simulink model "AttitudeControlSim"  (R2024b)
settings: Solver=VariableStepAuto  StartTime=0.0  StopTime=1000  RelTol=1e-3
values from neighbouring files (symbols this model uses):
  A = RWSConfig(beta)    [RWSTiltAngleOptimisation.m]
  Js = 0.001    [RWSTiltAngleOptimisation.m]
  Kd = diag([20;20;24])    [RWSTiltAngleOptimisation.m]
  Kp = diag([10;10;12])    [RWSTiltAngleOptimisation.m]
  omega0 = 0    [RWSTiltAngleOptimisation.m]
undefined symbols (not defined in the file or in its folder): orb, sat
libraries: aerolibutil x3, matrix_library x2, sharedutil x1
settings Model: PacingRate=2  Creator=Ameya  LastModifiedBy=Ameya

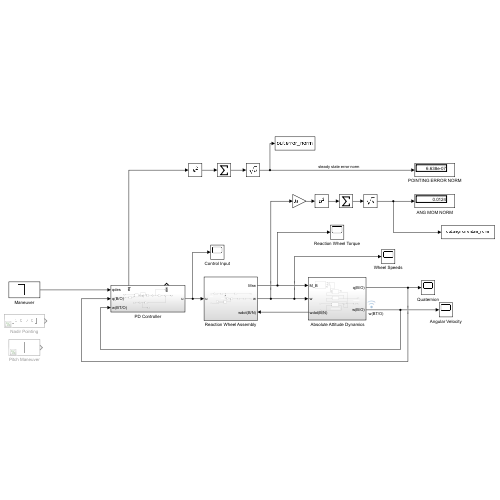
[thumbnail: Simulink's stored preview of the top-level diagram]
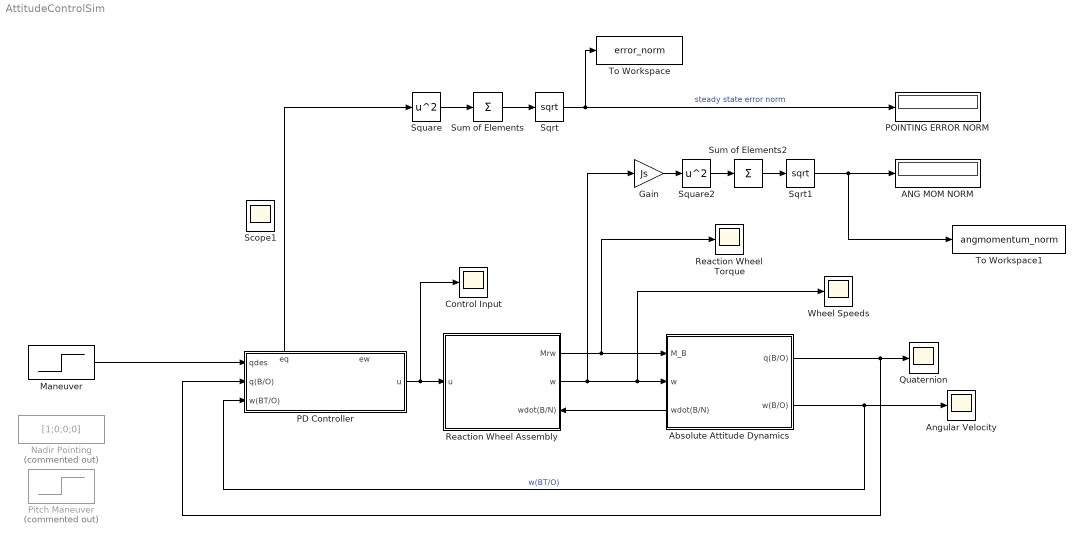
== system AttitudeControlSim ==
  " Absolute Attitude Dynamics" : Subsystem
      settings: PortSchema="{\"entries\":[{\"content\":{\"sides\":[{\"content\":{\"connectorIds\":[\"In1\",\"In2\",\"Out3\"]},\"type\":\"ConnectorPlacement.EquallySpacedRectSide\",\"uuid\":\"5cc1fa62-5eb8-4e37-8643-9896299a6aa0\"},{\"content\":{\"connectorIds\":[\"Out1\",\"Out2\"],\"side\":\"RIGHT\"},\"type\":\"ConnectorPlacement.EquallySpacedRectSide\",\"uuid\":\"f1722523-4fb3-4755-a040-6e35a0c45818\"},{\"content\":{\"side\":\"TOP\"},\"type\":\"ConnectorPlacement.EquallySpacedRectSide\",\"uuid\":\"c8585ddf-0cc3-42b7-bd60-482c1818a7a4\"}]},\"type\":\"ConnectorPlacement.EquallySpacedConnector\",\"uuid\":\"15ebf4a1-1e12-47bd-82f1-7178c1be1ccf\"}],\"packageUris\":[\"http://schema.mathworks.com/mf0/Connector/R2020b\"],\"version\":\"1.0\"}"
  ANG MOM NORM : Display
  Angular Velocity : Scope
  Control Input : Scope
  Gain : Gain  Gain=Js
  Maneuver : Step  Time=5  Before=[1;0;0;0]  After=[0.9893;0.07893;0.09406;0.07893]  SampleTime=0
  Nadir Pointing : Constant  Commented=on  Value=[1;0;0;0]
  PD Controller : Subsystem
      settings: PortSchema="{\"entries\":[{\"content\":{\"sides\":[{\"content\":{\"connectorIds\":[\"In1\",\"In2\",\"In3\"]},\"type\":\"ConnectorPlacement.EquallySpacedRectSide\",\"uuid\":\"a46acad7-148c-4190-8160-1acb5439ed3f\"},{\"content\":{\"connectorIds\":[\"Out1\"],\"side\":\"RIGHT\"},\"type\":\"ConnectorPlacement.EquallySpacedRectSide\",\"uuid\":\"677782f5-c393-46c5-8dbb-c8a019f7e2a6\"},{\"content\":{\"connectorIds\":[\"Out2\",\"Out3\"],\"side\":\"TOP\"},\"type\":\"ConnectorPlacement.EquallySpacedRectSide\",\"uuid\":\"40cea264-8167-4aef-b4a8-0c746fd0cc26\"}]},\"type\":\"ConnectorPlacement.EquallySpacedConnector\",\"uuid\":\"6b37b8a2-a3d8-44f8-9256-f1896837436e\"}],\"packageUris\":[\"http://schema.mathworks.com/mf0/Connector/R2020b\"],\"version\":\"1.0\"}"
  POINTING ERROR NORM : Display
  Pitch Maneuver : Step  Commented=on  Time=5  Before=[1;0;0;0]  After=[cos(deg2rad(2.5));0;0;sin(deg2rad(2.5))]  SampleTime=0
  Quaternion : Scope
  Reaction Wheel Assembly : Subsystem
      settings: PortSchema="{\"entries\":[{\"content\":{\"sides\":[{\"content\":{\"connectorIds\":[\"In1\"]},\"type\":\"ConnectorPlacement.EquallySpacedRectSide\",\"uuid\":\"57a5e211-d888-47e5-a410-d74309a415f6\"},{\"content\":{\"connectorIds\":[\"Out1\",\"Out2\",\"In2\"],\"side\":\"RIGHT\"},\"type\":\"ConnectorPlacement.EquallySpacedRectSide\",\"uuid\":\"0d6436a4-96ad-4035-90dd-04c735a462cf\"},{\"content\":{\"side\":\"TOP\"},\"type\":\"ConnectorPlacement.EquallySpacedRectSide\",\"uuid\":\"eefef678-a1c2-433e-9ac3-082bc8edd153\"}]},\"type\":\"ConnectorPlacement.EquallySpacedConnector\",\"uuid\":\"6794547d-8daf-40ab-9bc3-64f70f726c2c\"}],\"packageUris\":[\"http://schema.mathworks.com/mf0/Connector/R2020b\"],\"version\":\"1.0\"}"
  Reaction Wheel Torque : Scope
  Sqrt : Sqrt
  Sqrt1 : Sqrt
  Square : Math  Operator=square
  Square2 : Math  Operator=square
  Sum of Elements : Sum  Inputs=+
  Sum of Elements2 : Sum  Inputs=+
  To Workspace : ToWorkspace  VariableName=error_norm  SaveFormat=Timeseries  SampleTime=-1
  To Workspace1 : ToWorkspace  VariableName=angmomentum_norm  SaveFormat=Timeseries  SampleTime=-1
  Wheel Speeds : Scope
  Scope1 : Scope
  wires:
  Reaction Wheel Assembly/2(w) -> Wheel Speeds/1, " Absolute Attitude Dynamics"/2(w), Gain/1
  " Absolute Attitude Dynamics"/3(wdot(B/N)) -> Reaction Wheel Assembly/2(wdot(B/N))
  " Absolute Attitude Dynamics"/2(w(B/O)) -> PD Controller/3(w(BT/O)), Angular Velocity/1  "w(BT/O)"
  " Absolute Attitude Dynamics"/1(q(B/O)) -> Quaternion/1, PD Controller/2(q(B/O))
  PD Controller/1(u) -> Control Input/1, Reaction Wheel Assembly/1(u)
  Reaction Wheel Assembly/1(Mrw) -> Reaction Wheel Torque/1, " Absolute Attitude Dynamics"/1(M_B)
  PD Controller/2(eq) -> Square/1
  Square/1 -> Sum of Elements/1
  Sum of Elements/1 -> Sqrt/1
  Square2/1 -> Sum of Elements2/1
  Gain/1 -> Square2/1
  Sum of Elements2/1 -> Sqrt1/1
  Sqrt/1 -> To Workspace/1, POINTING ERROR NORM/1  "steady state error norm"
  Sqrt1/1 -> To Workspace1/1, ANG MOM NORM/1
  Maneuver/1 -> PD Controller/1(qdes)

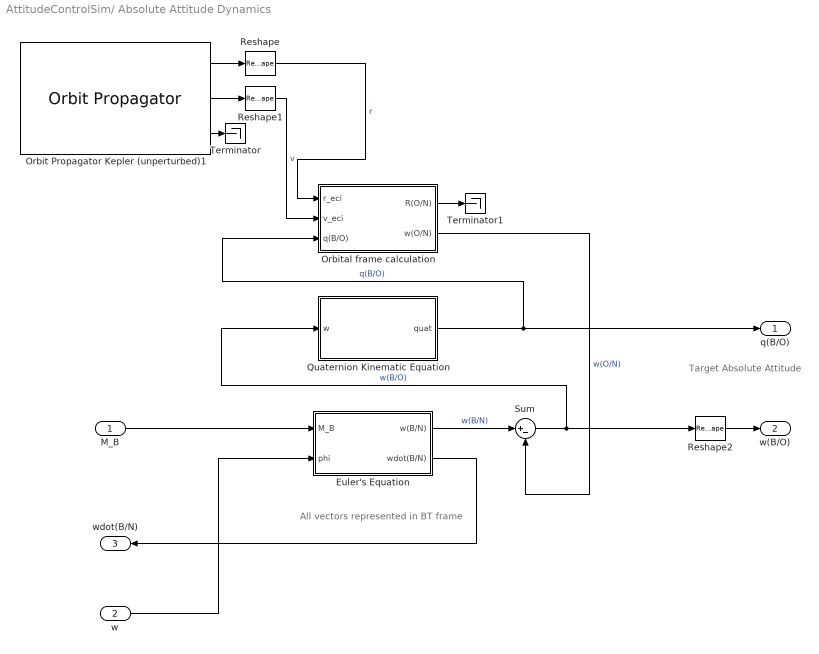
== system AttitudeControlSim/ Absolute Attitude Dynamics ==
  note: Target Absolute Attitude
  note: All vectors represented in BT frame
  M_B : Inport
  w : Inport  Port=2
  Euler's Equation : Subsystem
  Orbit Propagator Kepler (unperturbed)1 : OrbitPropagator  accelIn=on  startDate=start_time  semiMajorAxis=orb.a  eccentricity=orb.e  inclination=orb.i  raan=orb.RAAN  argPeriapsis=orb.w  trueAnomaly=orb.ta  inertialPosition=[3649700.0 3308200.0 -4676600.0]  inertialVelocity=[-2750.8 6666.4 2573.4]  fixedPosition=[-4142689.0 -2676864.7 -4669861.6]  fixedVelocity=[1452.7 -6720.7 2568.1]  gravityModel=Oblate ellipsoid (J2)  customR=3396200  customMu=4.305e13  customJ2=1.0826269e-03  customOmega=4.06125949e-3  angleUnits=Radians
  Orbital frame calculation : Subsystem
  Quaternion Kinematic Equation : Subsystem
  Reshape : Reshape  OutputDimensionality=Column vector (2-D)
  Reshape1 : Reshape  OutputDimensionality=Column vector (2-D)
  Reshape2 : Reshape  OutputDimensionality=Column vector (2-D)
  Sum : Sum  Inputs=|+-
  Terminator : Terminator
  Terminator1 : Terminator
  q(B/O) : Outport
  w(B/O) : Outport  Port=2
  wdot(B/N) : Outport  Port=3
  wires:
  Orbit Propagator Kepler (unperturbed)1/2 -> Reshape1/1
  Reshape/1 -> Orbital frame calculation/1(r_eci)  "r"
  Sum/1 -> Reshape2/1, Quaternion Kinematic Equation/1(w)  "w(B/O)"
  Reshape1/1 -> Orbital frame calculation/2(v_eci)  "v"
  M_B/1 -> Euler's Equation/1(M_B)
  Orbit Propagator Kepler (unperturbed)1/1 -> Reshape/1
  Orbital frame calculation/2(w(O/N)) -> Sum/2  "w(O/N)"
  Orbital frame calculation/1(R(O/N)) -> Terminator1/1
  Euler's Equation/1(w(B/N)) -> Sum/1  "w(B/N)"
  Quaternion Kinematic Equation/1(quat) -> q(B/O)/1, Orbital frame calculation/3(q(B/O))  "q(B/O)"
  Orbit Propagator Kepler (unperturbed)1/3 -> Terminator/1
  Euler's Equation/2(wdot(B/N)) -> wdot(B/N)/1
  w/1 -> Euler's Equation/2(phi)
  Reshape2/1 -> w(B/O)/1

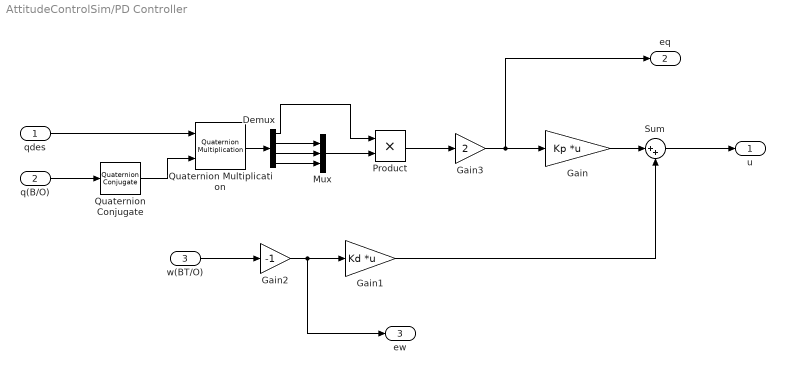
== system AttitudeControlSim/PD Controller ==
  qdes : Inport
  q(B/O) : Inport  Port=2
  w(BT/O) : Inport  Port=3
  Demux : Demux
  Gain : Gain  Gain=Kp  Multiplication=Matrix(K*u)
  Gain1 : Gain  Gain=Kd  Multiplication=Matrix(K*u)
  Gain2 : Gain  Gain=-1
  Gain3 : Gain  Gain=2
  Mux : Mux  Inputs=3
  Product : Product
  Quaternion Conjugate : aerolibutil/Quaternion Conjugate
  Quaternion Multiplication : aerolibutil/Quaternion Multiplication
  Sum : Sum  Inputs=|++
  u : Outport
  eq : Outport  Port=2
  ew : Outport  Port=3
  wires:
  qdes/1 -> Quaternion Multiplication/1
  q(B/O)/1 -> Quaternion Conjugate/1
  Quaternion Conjugate/1 -> Quaternion Multiplication/2
  Gain/1 -> Sum/1
  w(BT/O)/1 -> Gain2/1
  Sum/1 -> u/1
  Quaternion Multiplication/1 -> Demux/1
  Demux/1 -> Product/1
  Product/1 -> Gain3/1
  Mux/1 -> Product/2
  Demux/2 -> Mux/1
  Demux/3 -> Mux/2
  Demux/4 -> Mux/3
  Gain2/1 -> ew/1, Gain1/1
  Gain1/1 -> Sum/2
  Gain3/1 -> eq/1, Gain/1

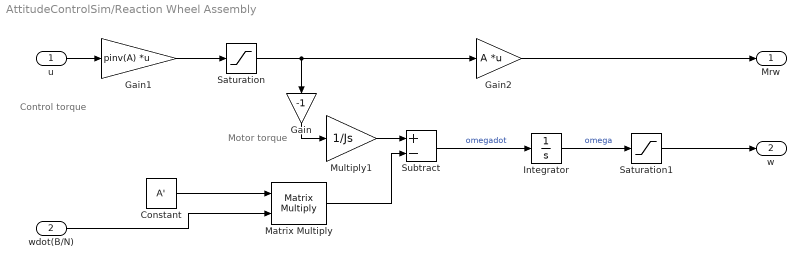
== system AttitudeControlSim/Reaction Wheel Assembly ==
  note: Control torque
  note: Motor torque
  u : Inport
  wdot(B/N) : Inport  Port=2
  Constant : Constant  Value=A'
  Gain : Gain  Gain=-1
  Gain1 : Gain  Gain=pinv(A)  Multiplication=Matrix(K*u)
  Gain2 : Gain  Gain=A  Multiplication=Matrix(K*u)
  Integrator : Integrator  InitialCondition=omega0
  Matrix Multiply : Product  Multiplication=Matrix(*)
  Multiply1 : Gain  Gain=1/Js
  Saturation : Saturate  UpperLimit=0.05  LowerLimit=-0.05
  Saturation1 : Saturate  UpperLimit=5000*2*pi/60  LowerLimit=-5000*2*pi/60
  Subtract : Sum  Inputs=+-
  Mrw : Outport
  w : Outport  Port=2
  wires:
  Subtract/1 -> Integrator/1  "omegadot"
  Integrator/1 -> Saturation1/1  "omega"
  Saturation/1 -> Gain2/1, Gain/1
  u/1 -> Gain1/1
  Multiply1/1 -> Subtract/1
  Matrix Multiply/1 -> Subtract/2
  Saturation1/1 -> w/1
  Gain/1 -> Multiply1/1
  Gain1/1 -> Saturation/1
  Gain2/1 -> Mrw/1
  Constant/1 -> Matrix Multiply/1
  wdot(B/N)/1 -> Matrix Multiply/2

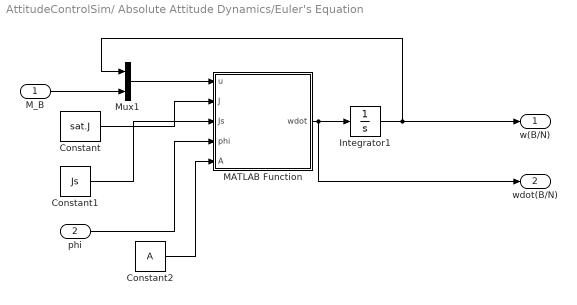
== system AttitudeControlSim/ Absolute Attitude Dynamics/Euler's Equation ==
  M_B : Inport
  phi : Inport  Port=2
  Constant : Constant  Value=sat.J
  Constant1 : Constant  Value=Js
  Constant2 : Constant  Value=A
  Integrator1 : Integrator  InitialCondition=sat.omegaBN
  MATLAB Function : MATLAB Function  TreatAsAtomicUnit=on
  Mux1 : Mux  Inputs=2
  w(B/N) : Outport
  wdot(B/N) : Outport  Port=2
  wires:
  M_B/1 -> Mux1/2
  MATLAB Function/1(wdot) -> wdot(B/N)/1, Integrator1/1
  Integrator1/1 -> Mux1/1, w(B/N)/1
  Mux1/1 -> MATLAB Function/1(u)
  Constant/1 -> MATLAB Function/2(J)
  Constant1/1 -> MATLAB Function/3(Js)
  phi/1 -> MATLAB Function/4(phi)
  Constant2/1 -> MATLAB Function/5(A)

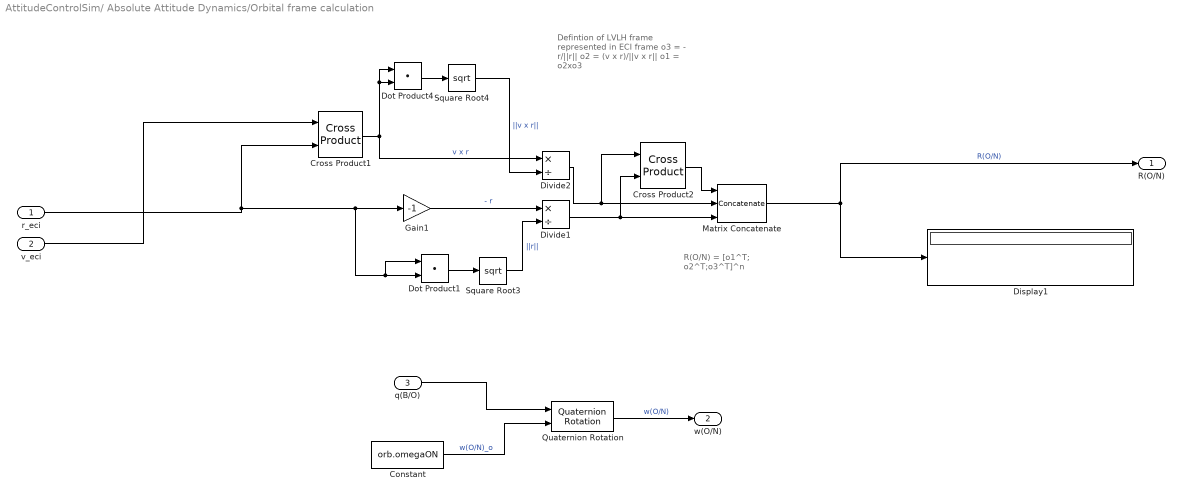
== system AttitudeControlSim/ Absolute Attitude Dynamics/Orbital frame calculation ==
  note: R(O/N) = [o1^T; o2^T;o3^T]^n
  note: Defintion of LVLH frame
      | represented in ECI frame
      | o3 = - r/||r||
      | o2 = (v x r)/||v x r||
      | o1 = o2xo3
  r_eci : Inport
  v_eci : Inport  Port=2
  q(B/O) : Inport  Port=3
  Constant : Constant  Value=orb.omegaON
  Cross Product1 : matrix_library/Cross Product
  Cross Product2 : matrix_library/Cross Product
  Display1 : Display
  Divide1 : Product  Inputs=*/
  Divide2 : Product  Inputs=*/
  Dot Product1 : DotProduct  OutDataTypeStr=Inherit: Inherit via internal rule
  Dot Product4 : DotProduct  OutDataTypeStr=Inherit: Inherit via internal rule
  Gain1 : Gain  Gain=-1
  Matrix Concatenate : Concatenate  NumInputs=3  Mode=Multidimensional array  ConcatenateDimension=2
  Quaternion Rotation : aerolibutil/Quaternion Rotation
  Square Root3 : Sqrt
  Square Root4 : Sqrt
  R(O/N) : Outport
  w(O/N) : Outport  Port=2
  wires:
  q(B/O)/1 -> Quaternion Rotation/1
  Quaternion Rotation/1 -> w(O/N)/1  "w(O/N)"
  Constant/1 -> Quaternion Rotation/2  "w(O/N)_o"
  Cross Product2/1 -> Matrix Concatenate/1
  Divide2/1 -> Cross Product2/1, Matrix Concatenate/2
  Cross Product1/1 -> Dot Product4/2, Dot Product4/1, Divide2/1  "v x r"
  r_eci/1 -> Cross Product1/2, Dot Product1/1, Dot Product1/2, Gain1/1
  Gain1/1 -> Divide1/1  "- r"
  Square Root3/1 -> Divide1/2  "||r||"
  Square Root4/1 -> Divide2/2  "||v x r||"
  Dot Product1/1 -> Square Root3/1
  v_eci/1 -> Cross Product1/1
  Matrix Concatenate/1 -> Display1/1, R(O/N)/1  "R(O/N)"
  Divide1/1 -> Cross Product2/2, Matrix Concatenate/3
  Dot Product4/1 -> Square Root4/1

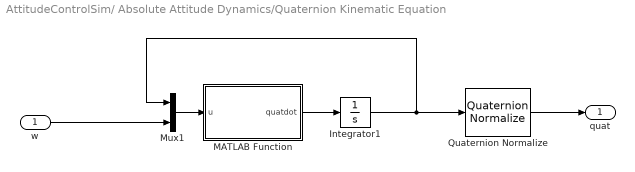
== system AttitudeControlSim/ Absolute Attitude Dynamics/Quaternion Kinematic Equation ==
  w : Inport
  Integrator1 : Integrator  InitialCondition=sat.quat
  MATLAB Function : MATLAB Function  TreatAsAtomicUnit=on
  Mux1 : Mux  Inputs=2
  Quaternion Normalize : sharedutil/Quaternion Normalize  aMode=aMode
  quat : Outport
  wires:
  Mux1/1 -> MATLAB Function/1(u)
  Integrator1/1 -> Quaternion Normalize/1, Mux1/1
  MATLAB Function/1(quatdot) -> Integrator1/1
  w/1 -> Mux1/2
  Quaternion Normalize/1 -> quat/1

== matlab function AttitudeControlSim/ Absolute Attitude Dynamics/Euler's Equation/MATLAB Function ==
  data: u input; wdot output; J input; Js input; phi input; A input
function wdot = EulersEOM(u,J,Js,phi,A)
    w = u(1:3);
    m = u(4:6);
    wdot = J\(-cross(w,(J*w + A*Js*phi))+m);
end

== matlab function AttitudeControlSim/ Absolute Attitude Dynamics/Quaternion Kinematic Equation/MATLAB Function ==
  data: u input; quatdot output
function quatdot = quatKinematics(u)
    quat = u(1:4);
    p = u(5);
    q = u(6);
    r = u(7);
    quatdot = 0.5*[0,-p,-q,-r;
                p,0,r,-q;
                q,-r,0,p;
                r,q,-p,0]*quat;
end
